simulink model "Recon"  (R2017b)
settings: Solver=FixedStepDiscrete  StartTime=0.0  StopTime=0.4  RelTol=1e-3
libraries: dspsigops x2, dsparch4 x1
settings Model: Creator=julied  LastModifiedBy=agarwal
settings SolverCC: AutoInsertRateTranBlk=on
settings DataIOCC: LimitDataPoints=on  SaveOutput=off  SignalLogging=off  SaveTime=off
settings OptimizationCC: LifeSpan=inf
settings DebuggingCC: AlgebraicLoopMsg=error  SingleTaskRateTransMsg=error  AllowSymbolicDim=off  SFUnexpectedBacktrackingDiag=warning  SFNoUnconditionalDefaultTransitionDiag=warning  SFExecutionAtInitializationDiag=none
settings CodeAppCC: StateflowObjectComments=on
settings GRTTargetCC: TargetLangStandard=C89/C90 (ANSI)  GeneratePreprocessorConditionals=Disable all

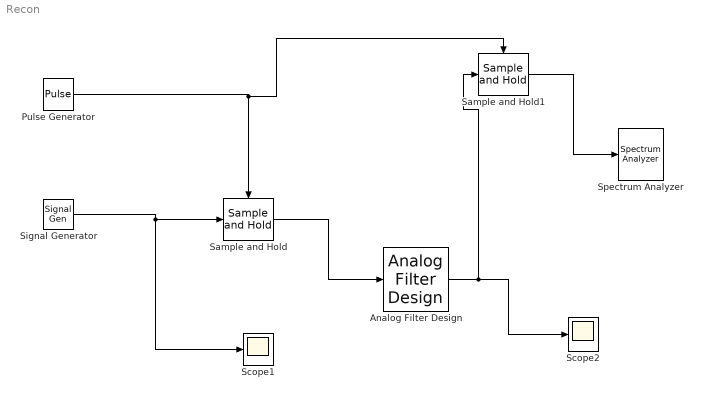
== system Recon ==
  Analog Filter Design : dsparch4/Analog Filter Design  method=Butterworth  filttype=Lowpass  N=8  Wlo=2*pi*250  Whi=80  Rp=2  Rs=40
  Pulse Generator : DiscretePulseGenerator  PulseType=Time based  Period=1/1000  PulseWidth=50  SampleTime=1/800
  Sample and Hold : dspsigops/Sample and Hold  trig=Rising edge  initCond=0  latchinput=off
  Sample and Hold1 : dspsigops/Sample and Hold  trig=Rising edge  initCond=0  latchinput=off
  Scope1 : Scope
  Scope2 : Scope
  Signal Generator : SignalGenerator  Amplitude=5  Frequency=200
  Spectrum Analyzer : SpectrumAnalyzer
  wires:
  Pulse Generator/1 -> Sample and Hold1/Trigger, Sample and Hold/Trigger
  Signal Generator/1 -> Scope1/1, Sample and Hold/1
  Sample and Hold/1 -> Analog Filter Design/1
  Analog Filter Design/1 -> Sample and Hold1/1, Scope2/1
  Sample and Hold1/1 -> Spectrum Analyzer/1
